simulink model "lead_controller"  (R2019b)
settings: Solver=FixedStepAuto  StartTime=0.0  StopTime=10.0  FixedStep=0.01  RelTol=1e-3
values from neighbouring files (symbols this model uses):
  alpha = (1-sin(phi))/(1+sin(phi))    [setup_lead_controller.m]
undefined symbols (not defined in the file or in its folder): T
settings Model: Creator=suvo  LastModifiedBy=suvo

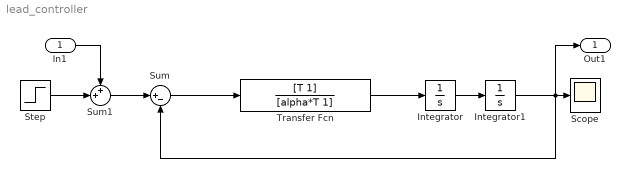
== system lead_controller ==
  In1 : Inport
  Integrator : Integrator
  Integrator1 : Integrator
  Scope : Scope
  Step : Step  SampleTime=0
  Sum : Sum  Inputs=|+-
  Sum1 : Sum  Inputs=++|
  Transfer Fcn : TransferFcn  Numerator=[T 1]  Denominator=[alpha*T 1]
  Out1 : Outport
  wires:
  Integrator/1 -> Integrator1/1
  Transfer Fcn/1 -> Integrator/1
  Integrator1/1 -> Out1/1, Sum/2, Scope/1
  Sum/1 -> Transfer Fcn/1
  Step/1 -> Sum1/2
  Sum1/1 -> Sum/1
  In1/1 -> Sum1/1
